simulink model "single_phase_half_bridge_inverter"  (R2021a)
settings: Solver=ode23tb  StartTime=0.0  StopTime=0.5  MaxStep=1e-4  RelTol=1e-3
values from neighbouring files (symbols this model uses):
  Ac = 1    [Inverter_parameters.m]
  Ar = ma*Ac    (= 0.5)    [Inverter_parameters.m]
  fc1 = mf1*f    (= 1000)    [Inverter_parameters.m]
  fc2 = mf2*f    (= 1150)    [Inverter_parameters.m]
  fr = 2*pi*f    (= 314.159265359)    [Inverter_parameters.m]
  L = X/(2*pi*f)    (= 0.0999493042617)    [Inverter_parameters.m]
  R = 100    [Inverter_parameters.m]
  t1 = alpha_new(1)*t/360    [selective_harmonic_elimination.m]
  t2 = alpha_new(2)*t/360    [selective_harmonic_elimination.m]
  to = 1e-9    (= 1e-09)    [selective_harmonic_elimination.m]
  Vin = 780    [Inverter_parameters.m]
libraries: spsRMSLib x5, simulink x3, spsCurrentMeasurementLib x2, spsDCVoltageSourceLib x2, spsIGBTDiodeLib x2, spsSeriesRLCBranchLib x1, spsVoltageMeasurementLib x1, spspowerguiLib x1
settings Model: Creator=HossamAladdin  LastModifiedBy=HossamAladdin
settings DataIOCC: ReturnWorkspaceOutputs=off

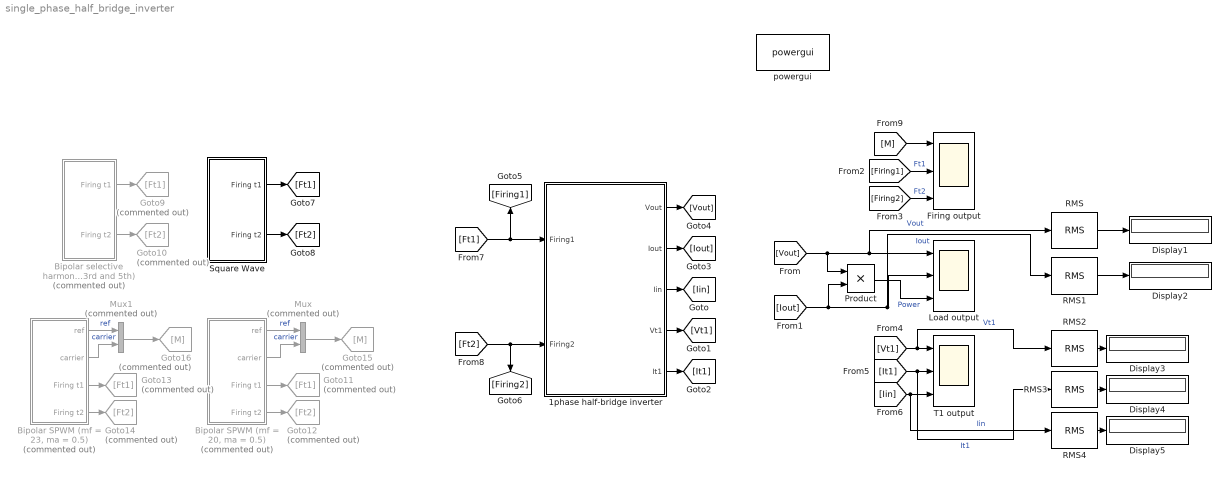
== system single_phase_half_bridge_inverter ==
  1phase half-bridge inverter : Subsystem
  "Bipolar SPWM (mf = 20, ma = 0.5)" : Subsystem  Commented=on
  "Bipolar SPWM (mf = 23, ma = 0.5)" : Subsystem  Commented=on
  Bipolar selective harmonic elimination (eliminate 3rd and 5th) : Subsystem  Commented=on
  Display{1..5} (5 alike) : Display
  Firing output : Scope  NumInputPorts=3
  Goto10 : Goto  Commented=on  GotoTag=Ft2
  Goto11 : Goto  Commented=on  GotoTag=Ft1
  Goto12 : Goto  Commented=on  GotoTag=Ft2
  Goto13 : Goto  Commented=on  GotoTag=Ft1
  Goto14 : Goto  Commented=on  GotoTag=Ft2
  Goto15 : Goto  Commented=on  GotoTag=M
  Goto16 : Goto  Commented=on  GotoTag=M
  Goto9 : Goto  Commented=on  GotoTag=Ft1
  Load output : Scope  NumInputPorts=3
  Mux : Mux  Commented=on  Inputs=2
  Mux1 : Mux  Commented=on  Inputs=2
  Product : Product
  RMS{,1..4} (5 alike) : spsRMSLib/RMS  TrueRMS=on  Freq=50  RMSInit=0  Ts=0
  Square Wave : Subsystem
  T1 output : Scope  NumInputPorts=3
  powergui : spspowerguiLib/powergui  Priority=1  SimulationMode=Discrete  SampleTime=1e-6  frequency=60  Iterations=50  frequencyindice=0  Pbase=100e6  ErrMax=1e-4  UnitsV=kV  UnitsW=MW  buscounter=0  FunctionMessages=off  echomessages=off  EnableUseOfTLC=off  CurrentSourceSwitches=off  DisableSnubberDevices=off  DisableRonSwitches=off  DisableVfSwitches=off  DisplayEquations=off  AutomaticDiscreteSolvers=off  SolverType=Tustin/Backward Euler (TBE)  Interpol=off  ExternalGateDelay=off  methode=off  Ts=100  x0status=blocks  SPID=on  SwTol=0  HookPort=off  NonlinearTolerance=1e-4  nMaxIteration=100  ContinueOnMaxIteration=off  RestoreLinks=warning  ResistiveCurrentMeasurement=off  Frange=[0:2:500]  Ylog=off  Xlog=on  ShowGrid=off  save=off  variable=ZData  structure=0  ZoomFFT=off  StartTime=0.0  cycles=1  DisplayStyle=1  fundamental=60  FreqAxis=off  MaxFrequency=1000  frequencyindicesteady=1  RmsSteady=1  display=off
  wires:
  [Firing1] -> Firing output/2  "Ft1"
  1phase half-bridge inverter/1(Vout) -> [Vout]
  [Iin] -> RMS4/1, T1 output/3  "Iin"
  [It1] -> RMS3/1, T1 output/2  "It1"
  1phase half-bridge inverter/2(Iout) -> [Iout]
  1phase half-bridge inverter/3(Iin) -> [Iin]
  1phase half-bridge inverter/5(It1) -> [It1]
  Product/1 -> Load output/3  "Power"
  [Vout] -> RMS/1, Load output/1, Product/1  "Vout"
  1phase half-bridge inverter/4(Vt1) -> [Vt1]
  [Vt1] -> RMS2/1, T1 output/1  "Vt1"
  [Firing2] -> Firing output/3  "Ft2"
  Square Wave/1(Firing t1) -> [Ft1]
  Square Wave/2(Firing t2) -> [Ft2]
  Bipolar selective harmonic elimination (eliminate 3rd and 5th)/2(Firing t2) -> Goto10/1
  Bipolar selective harmonic elimination (eliminate 3rd and 5th)/1(Firing t1) -> Goto9/1
  "Bipolar SPWM (mf = 20, ma = 0.5)"/4(Firing t2) -> Goto12/1
  "Bipolar SPWM (mf = 20, ma = 0.5)"/3(Firing t1) -> Goto11/1
  "Bipolar SPWM (mf = 23, ma = 0.5)"/3(Firing t1) -> Goto13/1
  "Bipolar SPWM (mf = 23, ma = 0.5)"/4(Firing t2) -> Goto14/1
  [Ft1] -> [Firing1], 1phase half-bridge inverter/1(Firing1)
  [Ft2] -> [Firing2], 1phase half-bridge inverter/2(Firing2)
  RMS/1 -> Display1/1
  RMS1/1 -> Display2/1
  [Iout] -> RMS1/1, Load output/2, Product/2  "Iout"
  RMS2/1 -> Display3/1
  RMS3/1 -> Display4/1
  RMS4/1 -> Display5/1
  [M] -> Firing output/1
  Mux/1 -> Goto15/1
  "Bipolar SPWM (mf = 20, ma = 0.5)"/1(ref) -> Mux/1  "ref"
  "Bipolar SPWM (mf = 20, ma = 0.5)"/2(carrier) -> Mux/2  "carrier"
  "Bipolar SPWM (mf = 23, ma = 0.5)"/2(carrier) -> Mux1/2  "carrier"
  "Bipolar SPWM (mf = 23, ma = 0.5)"/1(ref) -> Mux1/1  "ref"
  Mux1/1 -> Goto16/1

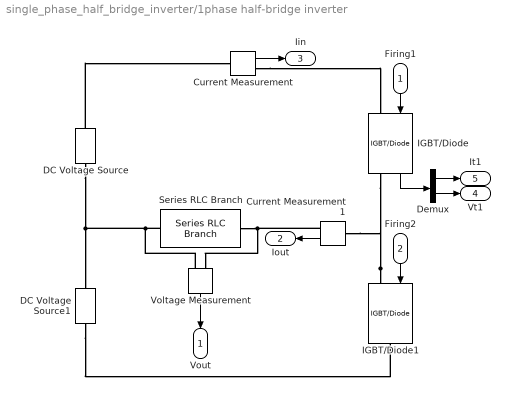
== system single_phase_half_bridge_inverter/1phase half-bridge inverter ==
  Firing1 : Inport
  Firing2 : Inport  Port=2
  Current Measurement : spsCurrentMeasurementLib/Current Measurement  PhasorSimulation=off  OutputType=Complex  PSBequivalent=0
  Current Measurement1 : spsCurrentMeasurementLib/Current Measurement  PhasorSimulation=off  OutputType=Complex  PSBequivalent=0
  DC Voltage Source : spsDCVoltageSourceLib/DC Voltage Source  Amplitude=Vin/2  Measurements=None
  DC Voltage Source1 : spsDCVoltageSourceLib/DC Voltage Source  Amplitude=Vin/2  Measurements=None
  Demux : Demux  Outputs=2
  IGBT/Diode : spsIGBTDiodeLib/IGBT//Diode  Ron=1e-3  Rs=1e5  Cs=inf  Measurements=on
  IGBT/Diode1 : spsIGBTDiodeLib/IGBT//Diode  Ron=1e-3  Rs=1e5  Cs=inf  Measurements=off
  Series RLC Branch : spsSeriesRLCBranchLib/Series RLC Branch  LConnTagsString=__new0  RConnTagsString=__new0  BranchType=RL  Resistance=R  Inductance=L  SetiL0=off  InitialCurrent=0  Capacitance=1e-6  Setx0=off  InitialVoltage=0  Measurements=None
  Voltage Measurement : spsVoltageMeasurementLib/Voltage Measurement  PhasorSimulation=off  OutputType=Complex  PSBequivalent=0
  Vout : Outport
  Iout : Outport  Port=2
  Iin : Outport  Port=3
  Vt1 : Outport  Port=4
  It1 : Outport  Port=5
  wires:
  IGBT/Diode/1 -> Demux/1
  Current Measurement1/1 -> Iout/1
  Current Measurement/1 -> Iin/1
  Firing1/1 -> IGBT/Diode/1
  Voltage Measurement/1 -> Vout/1
  Firing2/1 -> IGBT/Diode1/1
  Demux/2 -> Vt1/1
  Demux/1 -> It1/1
  connections:
  DC Voltage Source1/LConn1 -- IGBT/Diode1/RConn1
  Series RLC Branch/RConn1 -- Current Measurement1/RConn1 -- Voltage Measurement/LConn1
  Current Measurement/RConn1 -- IGBT/Diode/LConn1
  DC Voltage Source/RConn1 -- Current Measurement/LConn1
  Series RLC Branch/LConn1 -- Voltage Measurement/LConn2 -- DC Voltage Source1/RConn1 -- DC Voltage Source/LConn1
  IGBT/Diode1/LConn1 -- Current Measurement1/LConn1 -- IGBT/Diode/RConn1

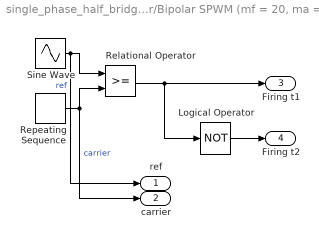
== system single_phase_half_bridge_inverter/Bipolar SPWM (mf = 20, ma = 0.5) ==
  Logical Operator : Logic  Operator=NOT  AllPortsSameDT=off  OutDataTypeStr=boolean
  Relational Operator : RelationalOperator  OutDataTypeStr=boolean  RndMeth=Simplest
  Repeating Sequence : simulink/Sources/Repeating Sequence  rep_seq_t=[0 (1/fc1)/4 (1/fc1)/2 (3/fc1)/4 (1/fc1)]  rep_seq_y=[0 Ac 0 -Ac 0]
  Sine Wave : Sin  Amplitude=Ar  Frequency=fr  SampleTime=0
  ref : Outport
  carrier : Outport  Port=2
  Firing t1 : Outport  Port=3
  Firing t2 : Outport  Port=4
  wires:
  Sine Wave/1 -> ref/1, Relational Operator/1  "ref"
  Relational Operator/1 -> Firing t1/1, Logical Operator/1
  Repeating Sequence/1 -> carrier/1, Relational Operator/2  "carrier"
  Logical Operator/1 -> Firing t2/1

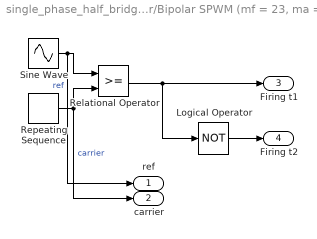
== system single_phase_half_bridge_inverter/Bipolar SPWM (mf = 23, ma = 0.5) ==
  Logical Operator : Logic  Operator=NOT  AllPortsSameDT=off  OutDataTypeStr=boolean
  Relational Operator : RelationalOperator  OutDataTypeStr=boolean  RndMeth=Simplest
  Repeating Sequence : simulink/Sources/Repeating Sequence  rep_seq_t=[0 (1/fc2)/4 (1/fc2)/2 (3/fc2)/4 (1/fc2)]  rep_seq_y=[0 Ac 0 -Ac 0]
  Sine Wave : Sin  Amplitude=Ar  Frequency=fr  SampleTime=0
  ref : Outport
  carrier : Outport  Port=2
  Firing t1 : Outport  Port=3
  Firing t2 : Outport  Port=4
  wires:
  Logical Operator/1 -> Firing t2/1
  Relational Operator/1 -> Logical Operator/1, Firing t1/1
  Repeating Sequence/1 -> carrier/1, Relational Operator/2  "carrier"
  Sine Wave/1 -> Relational Operator/1, ref/1  "ref"

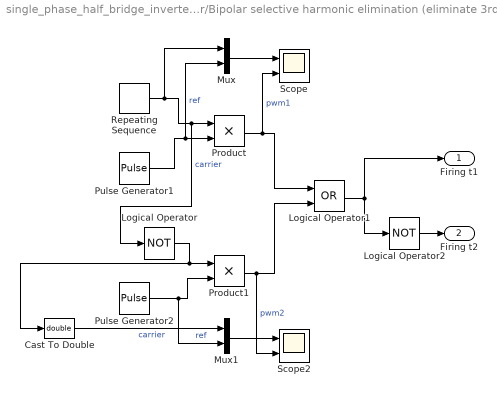
== system single_phase_half_bridge_inverter/Bipolar selective harmonic elimination (eliminate 3rd and 5th) ==
  Cast To Double : DataTypeConversion  OutDataTypeStr=double
  Logical Operator : Logic  Operator=NOT  AllPortsSameDT=off  OutDataTypeStr=boolean
  Logical Operator1 : Logic  Operator=OR  AllPortsSameDT=off  OutDataTypeStr=boolean
  Logical Operator2 : Logic  Operator=NOT  AllPortsSameDT=off  OutDataTypeStr=boolean
  Mux : Mux  Inputs=2
  Mux1 : Mux  Inputs=2
  Product : Product
  Product1 : Product
  Pulse Generator1 : DiscretePulseGenerator  PulseType=Time based  Period=t  PulseWidth=50
  Pulse Generator2 : DiscretePulseGenerator  PulseType=Time based  Period=t  PulseWidth=50  PhaseDelay=t/2
  Repeating Sequence : simulink/Sources/Repeating Sequence  rep_seq_t=[0 t1 t1+to t2 t2+to t/2-t2 t/2-t2+to t/2-t1 t/2-t1+to t/2]  rep_seq_y=[Ac Ac 0 0 Ac Ac 0 0 Ac Ac]
  Scope : Scope  NumInputPorts=2
  Scope2 : Scope  NumInputPorts=2
  Firing t1 : Outport
  Firing t2 : Outport  Port=2
  wires:
  Logical Operator/1 -> Product1/1, Cast To Double/1
  Repeating Sequence/1 -> Mux/1, Logical Operator/1, Product/1  "carrier"
  Product1/1 -> Scope2/2, Logical Operator1/2  "pwm2"
  Logical Operator2/1 -> Firing t2/1
  Logical Operator1/1 -> Firing t1/1, Logical Operator2/1
  Pulse Generator2/1 -> Mux1/2, Product1/2  "ref"
  Product/1 -> Scope/2, Logical Operator1/1  "pwm1"
  Pulse Generator1/1 -> Product/2, Mux/2  "ref"
  Mux/1 -> Scope/1
  Mux1/1 -> Scope2/1
  Cast To Double/1 -> Mux1/1  "carrier"

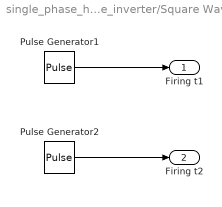
== system single_phase_half_bridge_inverter/Square Wave ==
  Pulse Generator1 : DiscretePulseGenerator  PulseType=Time based  Period=t  PulseWidth=50
  Pulse Generator2 : DiscretePulseGenerator  PulseType=Time based  Period=t  PulseWidth=50  PhaseDelay=t/2
  Firing t1 : Outport
  Firing t2 : Outport  Port=2
  wires:
  Pulse Generator1/1 -> Firing t1/1
  Pulse Generator2/1 -> Firing t2/1
